simulink model "controller14"  (R2023a)
settings: Solver=FixedStepAuto  StartTime=0.0  StopTime=mdl.rt  RelTol=1e-3
values from neighbouring files (symbols this model uses):
  archived_Eul_XYZ = rst_Eul_XYZ.signals.values    [s4_run.m]    (also in step4_run_v1.m)
  archived_p_raw = rst_p_raw.signals.values    [s4_run.m]    (also in step4_run_v1.m)
  ctr = make_ext_tor_observer(rsim, mdl, ctr)    [s1_setup.m]    (also in setup_controller_with_functions.m = make_controller(); step1_setup.m; step1_setup_v1.m)
  ctr2 = ctr    [s1_setup.m]    (also in step1_setup.m; step1_setup_v1.m)
  lut = gen_lut    [s1_setup.m]    (also in thrust2voltage_lut_20230809.mat = ; thrust2voltage_lut_20230829.mat = )
  mdl = make_model(mdl,rsim)    [s1_setup.m]    (also in setup_controller_with_functions.m = make_model(flight_time); step1_setup.m; step1_setup_v1.m = make_model(flight_time,rsim))
  rbt = make_robot    [s1_setup.m]    (also in setup_controller_with_functions.m = make_robot(); step1_setup.m; step1_setup_v1.m)
  rbt2 = rbt    [s1_setup.m]    (also in step1_setup.m; step1_setup_v1.m)
  rsim = make_robot_simulation()    [setup_controller_with_functions.m]    (also in step1_setup_v1.m = make_simulation(rbt,mdl,rsim))
  som = make_somersault(mdl, rsim)    [s1_setup.m]    (also in step1_setup.m = make_somersault(mdl))
  traj = make_trajectory(ctr, mdl, rsim)    [s1_setup.m]    (also in step1_setup.m)
undefined symbols (not defined in the file or in its folder): DiscIntNeverNeededParam, Standard_Devices, UDP_Protocol
libraries: simulink x27, dspfdesign x7, robotcorelib x6, sldrtlib x4, slrealtimeloglib x1, shared6dof x1, dspsrcs4 x1, uavutilslib x1
(part 1 of 3)
settings Model: SimulationMode=external  ExtModeTrigDuration=5000000  Creator=SMRL  LastModifiedBy=SMRL
settings HardwareCC: ProdBitPerLong=64  ProdHWDeviceType=Intel->x86-64 (Linux 64)
settings RTWCC: Description=Simulink Desktop Real-Time  SystemTargetFile=sldrt.tlc  TemplateMakefile=sldrt.tmf  RTWCompilerOptimization=on
settings CodeAppCC: MaxIdLength=95
settings SimulinkDesktopRealTimeCC: TargetLibSuffix=_sldrt.a  TargetPreCompLibLocation=C:\Program Files\MATLAB\R2023a\toolbox\sldrt\lib\win64

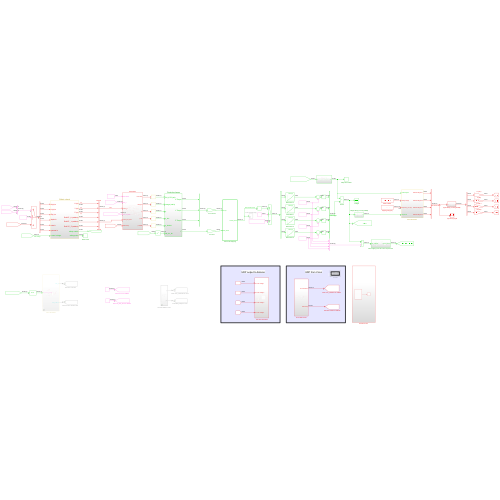
[thumbnail: Simulink's stored preview of the top-level diagram]
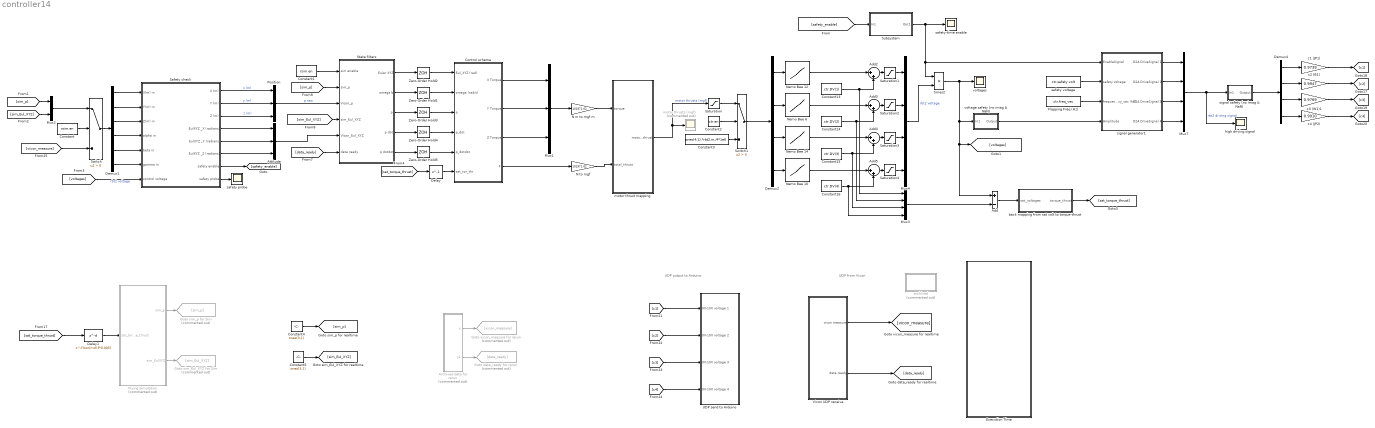
== system controller14 ==
  note: UDP output to Arduino
  note: UDP from Vicon
  Add : Sum  Inputs=+-
  Add{2..5} (4 alike) : Sum  Inputs=|++
  Archived data for rerun : Subsystem  Commented=on
  Attitude : Mux  Inputs=3
  Constant : Constant  Value=rsim.en
  Constant1 : Constant  Value=rsim.en
  Constant13 : Constant  Value=ctr.DV(1)
  Constant14 : Constant  Value=ctr.DV(2)
  Constant15 : Constant  Value=ctr.DV(3)
  Constant16 : Constant  Value=ctr.DV(4)
  Constant2 : Constant  Value=ctr.en
  Constant3 : Constant  Value=ones(4,1).*rbt2.m./4*1e6
  Constant4 : Constant  Value=ones(3,1)
  Constant5 : Constant  Value=ones(3,1)
  Control scheme : Subsystem
  Delay : Delay  DelayLength=1  InitialCondition=zeros(4,1)
  Delay1 : Delay  DelayLength=floor(mdl.f*0.005)  InitialCondition=zeros(4,floor(mdl.f*0.005))  SampleTime=mdl.T
  Demux1 : Demux  Outputs=6
  Demux2 : Demux
  Demux4 : Demux
  Execution Time : Subsystem
  Flapping Freq (Hz) : Constant  Value=ctr.freq_vec  VectorParams1D=off  SampleTime=mdl.T_high
  Flying Simulation : Subsystem  Commented=on
  Goto data_ready for rerun : Goto  Commented=on  GotoTag=data_ready
  Goto sim_Eul_XYZ for Sim : Goto  Commented=on  GotoTag=sim_Eul_XYZ
  Goto sim_p for Sim : Goto  Commented=on  GotoTag=sim_p
  Goto vicon_measure for rerun : Goto  Commented=on  GotoTag=vicon_measure
  Mux1 : Mux  Inputs=3
  Mux2 : Mux  Inputs=2
  Mux3 : Mux
  Mux4 : Mux
  Mux7 : Mux
  N m to mgf m : Gain  Gain=101971.62
  N to mgf : Gain  Gain=101971.62
  Nemo Bee 10 : Lookup_n-D  NumberOfTableDimensions=1  BreakpointsForDimension1=lut.T4  Table=lut.v4  InternalRulePriority=Speed  RndMeth=Simplest
  Nemo Bee 12 : Lookup_n-D  NumberOfTableDimensions=1  BreakpointsForDimension1=lut.T1  Table=lut.v1  InternalRulePriority=Speed  RndMeth=Simplest
  Nemo Bee 14 : Lookup_n-D  NumberOfTableDimensions=1  BreakpointsForDimension1=lut.T3  Table=lut.v3  InternalRulePriority=Speed  RndMeth=Simplest
  Nemo Bee 6 : Lookup_n-D  NumberOfTableDimensions=1  BreakpointsForDimension1=lut.T2  Table=lut.v2  InternalRulePriority=Speed  RndMeth=Simplest
  Position : Mux  Inputs=3
  Safety check : Subsystem  SystemSampleTime=mdl.T
  Saturation : Saturate  UpperLimit=1000  LowerLimit=0
  Saturation1 : Saturate  UpperLimit=ctr.safety.volt(1)  LowerLimit=0
  Saturation2 : Saturate  UpperLimit=ctr.safety.volt(2)  LowerLimit=0
  Saturation3 : Saturate  UpperLimit=ctr.safety.volt(3)  LowerLimit=0
  Saturation4 : Saturate  UpperLimit=ctr.safety.volt(4)  LowerLimit=0
  State filters : Subsystem
  Subsystem : Subsystem
  Switch : Switch  Criteria=u2 > Threshold  SaturateOnIntegerOverflow=off  InputSameDT=off
  Switch1 : Switch  Criteria=u2 > Threshold  SaturateOnIntegerOverflow=off  InputSameDT=off
  UDP send to Arduino : Subsystem
  Vicon UDP receive : Subsystem
  Zero-Order Hold{1..5} (5 alike) : ZeroOrderHold  SampleTime=mdl.T
  archived : Subsystem  Commented=on
  back mapping from sat volt to torque-thrust : Subsystem
  c1 (JP1) : Gain  Gain=0.9739
  c2 (B1) : Gain  Gain=0.9947
  c3 (W1)1 : Gain  Gain=0.9769
  c4 (JP2) : Gain  Gain=0.9910
  high driving signal : Scope
  motor thrust mapping : MATLAB Function  TreatAsAtomicUnit=on  SystemSampleTime=mdl.T
  motor thrusts (mgf) : Scope  Commented=on
  safety probe : Scope
  safety voltage : Constant  Value=ctr.safety.volt  SampleTime=mdl.T_high
  safety-time enable : Scope
  signal generator1 : Subsystem  SystemSampleTime=mdl.T_high
  signal safety (no imag & NaN) : Subsystem
  times2 : Product  RndMeth=Zero
  voltage safety (no imag & NaN) : Subsystem
  voltages : Scope
  wires:
  c3 (W1)1/1 -> [c3]
  c4 (JP2)/1 -> [c4]
  safety voltage/1 -> signal generator1/2(safety voltage)
  Demux4/4 -> c4 (JP2)/1
  signal safety (no imag & NaN)/1(Output) -> Demux4/1
  Safety check/3(Z (m)) -> Position/3  "z (m)"
  Demux4/3 -> c3 (W1)1/1
  Demux4/2 -> c2 (B1)/1
  voltage safety (no imag & NaN)/1(Output) -> signal generator1/4(Amplitude)
  Demux1/4 -> Safety check/4(alpha in)
  Safety check/2(Y (m)) -> Position/2  "y (m)"
  Saturation1/1 -> Mux4/1
  Saturation3/1 -> Mux4/3
  motor thrust mapping/1(motors_thrust) -> Saturation/1, motor thrusts (mgf)/1  "motor thrusts (mgf)"
  Demux4/1 -> c1 (JP1)/1
  Saturation2/1 -> Mux4/2
  Saturation4/1 -> Mux4/4
  Demux1/3 -> Safety check/3(Z(m) in)
  Demux1/2 -> Safety check/2(Y(m) in)
  signal generator1/1(D2A DriveSignal 1) -> Mux7/1
  Safety check/1(X (m)) -> Position/1  "x (m)"
  Mux7/1 -> signal safety (no imag & NaN)/1(In1), high driving signal/1  "rbt2 driving signal"
  c2 (B1)/1 -> [c2]
  Demux1/1 -> Safety check/1(X(m) in)
  c1 (JP1)/1 -> [c1]
  Demux1/6 -> Safety check/6(gamma in)
  signal generator1/2(D2A DriveSignal 2) -> Mux7/2
  signal generator1/3(D2A DriveSignal 3) -> Mux7/3
  Demux1/5 -> Safety check/5(beta in)
  Mux4/1 -> times2/2  "rbt2 voltage"
  Flapping Freq (Hz)/1 -> signal generator1/3(frequency_vec (hz))
  signal generator1/4(D2A DriveSignal 4) -> Mux7/4
  Safety check/6(EulXYZ _Z (radians)) -> Attitude/3
  Safety check/5(EulXYZ _Y (radians)) -> Attitude/2
  Safety check/4(EulXYZ _X (radians)) -> Attitude/1
  Vicon UDP receive/1(vicon measure) -> [vicon_measure]
  Vicon UDP receive/2(data ready) -> [data_ready]
  [c1] -> UDP send to Arduino/1(0V-10V voltage 1)
  [c2] -> UDP send to Arduino/2(0V-10V voltage 2)
  [c3] -> UDP send to Arduino/3(0V-10V voltage 3)
  [c4] -> UDP send to Arduino/4(0V-10V voltage 4)
  Safety check/7(safety enable) -> [safety_enable]
  Control scheme/1(X Torque) -> Mux1/1
  Control scheme/2(Y Torque) -> Mux1/2
  Control scheme/3(Z Torque) -> Mux1/3
  [sat_torque_thrust] -> Delay1/1
  Flying Simulation/2(sim_EulXYZ) -> Goto sim_Eul_XYZ for Sim/1
  Flying Simulation/1(sim_p) -> Goto sim_p for Sim/1
  [sim_p] -> Mux2/1
  [sim_Eul_XYZ] -> Mux2/2
  Constant/1 -> Switch/2
  Mux2/1 -> Switch/1
  [vicon_measure] -> Switch/3
  Switch/1 -> Demux1/1
  State filters/1(Euler XYZ) -> Zero-Order Hold2/1
  State filters/2(omega b) -> Zero-Order Hold1/1
  [sim_p] -> State filters/2(sim_p)
  [data_ready] -> State filters/6(data ready)
  State filters/3("p ") -> Zero-Order Hold3/1
  State filters/4(p dot) -> Zero-Order Hold4/1
  Position/1 -> State filters/3(Vicon_p)  "p raw"
  Constant1/1 -> State filters/1(sim enable)
  Attitude/1 -> State filters/5(Vicon_Eul_XYZ)
  [sim_Eul_XYZ] -> State filters/4(sim_Eul_XYZ)
  Zero-Order Hold2/1 -> Control scheme/1(Eul_XYZ (rad))
  Zero-Order Hold1/1 -> Control scheme/2(omega (rad/s))
  Zero-Order Hold3/1 -> Control scheme/3(p)
  Zero-Order Hold4/1 -> Control scheme/4(p_dot)
  Zero-Order Hold5/1 -> Control scheme/5(p_dotdot)
  State filters/5(p dotdot) -> Zero-Order Hold5/1
  N m to mgf m/1 -> motor thrust mapping/1(torque)
  N to mgf/1 -> motor thrust mapping/2(total_thrust)
  Constant14/1 -> Mux3/2, Add3/2
  Constant15/1 -> Mux3/3, Add4/2
  Constant16/1 -> Mux3/4, Add5/2
  Nemo Bee 6/1 -> Add3/1
  Nemo Bee 14/1 -> Add4/1
  Nemo Bee 12/1 -> Add2/1
  Nemo Bee 10/1 -> Add5/1
  Constant13/1 -> Mux3/1, Add2/2
  Add3/1 -> Saturation2/1
  Add2/1 -> Saturation1/1
  Add4/1 -> Saturation3/1
  Add5/1 -> Saturation4/1
  Demux2/1 -> Nemo Bee 12/1
  Demux2/2 -> Nemo Bee 6/1
  Demux2/3 -> Nemo Bee 14/1
  Demux2/4 -> Nemo Bee 10/1
  Constant2/1 -> Switch1/2
  Saturation/1 -> Switch1/1
  Switch1/1 -> Demux2/1
  Constant3/1 -> Switch1/3
  times2/1 -> voltage safety (no imag & NaN)/1(In1), [voltages], Add/1, voltages/1
  Constant4/1 -> [sim_p]
  Constant5/1 -> [sim_Eul_XYZ]
  [voltages] -> Safety check/7(control voltage)  "rbt2 voltage"
  Archived data for rerun/1(y) -> Goto vicon_measure for rerun/1
  Archived data for rerun/2(y1) -> Goto data_ready for rerun/1
  Mux3/1 -> Add/2
  Add/1 -> back mapping from sat volt to torque-thrust/1(sat_voltages)
  back mapping from sat volt to torque-thrust/1(torque_thrust) -> [sat_torque_thrust]
  Control scheme/4(" F") -> N to mgf/1
  Mux1/1 -> N m to mgf m/1
  Subsystem/1(Out1) -> signal generator1/1(EnableSignal), times2/1, safety-time enable/1
  [safety_enable] -> Subsystem/1(In1)
  Safety check/8(safety probe) -> safety probe/1
  [sat_torque_thrust] -> Delay/1
  Delay/1 -> Control scheme/6(sat_tor_thr)
  Delay1/1 -> Flying Simulation/1(sat_torque_thrust)

== system controller14/Archived data for rerun ==
  MATLAB Function1 : MATLAB Function  TreatAsAtomicUnit=on
  MATLAB Function2 : MATLAB Function  TreatAsAtomicUnit=on
  Scope1 : Scope
  Scope2 : Scope
  Scope3 : Scope
  time1 : Subsystem
  y : Outport
  y1 : Outport  Port=2
  wires:
  MATLAB Function2/1(y) -> y/1, Scope1/1
  time1/1(index) -> Scope2/1, MATLAB Function2/1(t), MATLAB Function1/1(t)
  MATLAB Function1/1(y) -> y1/1, Scope3/1

== system controller14/Control scheme ==
  Eul_XYZ (rad) : Inport
  omega (rad/s) : Inport  Port=2
  p : Inport  Port=3
  p_dot : Inport  Port=4
  p_dotdot : Inport  Port=5
  sat_tor_thr : Inport  Port=6
  Coordinate Transformation Conversion : robotcorelib/Coordinate Transformation Conversion  InputRepresentation=Euler Angles  InputEulerSequence=XYZ  ShowTrVecInputPort=on  OutputRepresentation=Rotation Matrix  OutputEulerSequence=ZYX  ShowTrVecOutputPort=on  SimulateUsing=Interpreted execution
  Delay : Delay  DelayLength=1  InitialCondition=1
  Delay1 : Delay  DelayLength=1  InitialCondition=zeros(3,1)
  adaptive setpoint rd : MATLAB Function  TreatAsAtomicUnit=on  SystemSampleTime=mdl.T
  all states : Scope  NumInputPorts=4
  attitude and thrust controller : Subsystem
  observer : Subsystem  Commented=on
  p vs p_des : Scope  NumInputPorts=2
  saturation : MATLAB Function  TreatAsAtomicUnit=on
  time : Subsystem
  unsat thrust : Scope
  unsat torque : Scope  NumInputPorts=3
  X Torque : Outport
  Y Torque : Outport  Port=2
  Z Torque : Outport  Port=3
  " F" : Outport  Port=4
  wires:
  Eul_XYZ (rad)/1 -> Coordinate Transformation Conversion/1
  omega (rad/s)/1 -> all states/4, attitude and thrust controller/5(Omega)
  saturation/1(X_roll) -> X Torque/1
  saturation/2(Y_pitch) -> Y Torque/1
  saturation/3(Z_yaw) -> Z Torque/1
  saturation/4(Force) -> " F"/1
  attitude and thrust controller/4(F) -> saturation/4(F), unsat thrust/1
  adaptive setpoint rd/1(rd) -> p vs p_des/2, attitude and thrust controller/6(rd)  "rd"
  adaptive setpoint rd/2(rd_d) -> attitude and thrust controller/7(rd_d)
  adaptive setpoint rd/3(rd_dd) -> attitude and thrust controller/8(rd_dd)
  adaptive setpoint rd/4(rd_ddd) -> attitude and thrust controller/9(rd_ddd)
  adaptive setpoint rd/5(rd_dddd) -> attitude and thrust controller/10(rd_dddd)
  time/1(real times) -> adaptive setpoint rd/2(time)
  attitude and thrust controller/3(torque_z) -> saturation/3(z_yaw), unsat torque/3
  attitude and thrust controller/2(torque_y) -> saturation/2(y_pitch), unsat torque/2
  attitude and thrust controller/1(torque_x) -> unsat torque/1, saturation/1(x_roll)
  adaptive setpoint rd/7(id_out) -> Delay/1
  Delay/1 -> adaptive setpoint rd/4(id_in)
  Coordinate Transformation Conversion/1 -> all states/3, attitude and thrust controller/4(R)  "rotm"
  p_dot/1 -> all states/2, attitude and thrust controller/2(r_dot)
  p_dotdot/1 -> attitude and thrust controller/3(r_dotdot)
  p/1 -> adaptive setpoint rd/1(r), p vs p_des/1, attitude and thrust controller/1(r), all states/1
  adaptive setpoint rd/6(init_r_out) -> Delay1/1
  Delay1/1 -> adaptive setpoint rd/3(init_r_in)
  sat_tor_thr/1 -> attitude and thrust controller/11(sat_tor_thr)

== system controller14/Execution Time ==
  Execution Time : sldrtlib/Target Profiling/Execution Time  ShowTaskTimes=off
  high execution time : Scope
  wires:
  Execution Time/1 -> high execution time/1

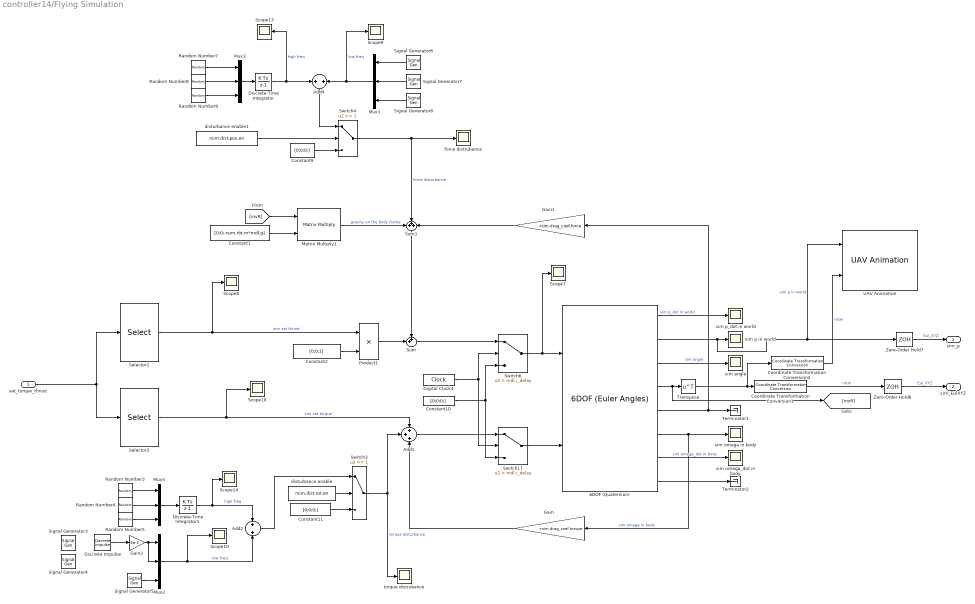
== system controller14/Flying Simulation ==
  sat_torque_thrust : Inport
  6DOF (Quaternion) : shared6dof/6DOF (Euler Angles)  units=Metric (MKS)  mtype=Fixed  rep=Quaternion  xme_0=rsim.p0  Vm_0=rsim.v0_b  eul_0=[rsim.Eul_XYZ.x rsim.Eul_XYZ.y rsim.Eul_XYZ.z]  pm_0=rsim.w0  mass_0=rsim.rbt.m  mass_e=0.5  mass_f=2.0  inertia=diag([rsim.rbt.ixx, rsim.rbt.iyy, rsim.rbt.izz])  inertia_e=eye(3)  inertia_f=2*eye(3)  k_quat=1.0  vre_flag=on  abi_flag=off  aMode=0  xme_statename=''  Vm_statename=''  eul_statename=''  quat_statename=''  pm_statename=''  mass_statename=''
      settings: LibrarySourceBlock=aerolib6dof2/6DOF (Quaternion)
  Add1 : Sum  Inputs=+++
  Add2 : Sum
  Add4 : Sum
  Constant1 : Constant  Value=[0;0;-rsim.rbt.m*mdl.g]
  Constant10 : Constant  Value=[0;0;0;]
  Constant11 : Constant  Value=[0;0;0;]
  Constant2 : Constant  Value=[0;0;1]
  Constant9 : Constant  Value=[0;0;0;]
  Coordinate Transformation Conversion1 : robotcorelib/Coordinate Transformation Conversion  InputRepresentation=Rotation Matrix  InputEulerSequence=XYZ  ShowTrVecInputPort=on  OutputRepresentation=Euler Angles  OutputEulerSequence=XYZ  ShowTrVecOutputPort=on  SimulateUsing=Interpreted execution
  Coordinate Transformation Conversion2 : robotcorelib/Coordinate Transformation Conversion  InputRepresentation=Rotation Matrix  InputEulerSequence=XYZ  ShowTrVecInputPort=on  OutputRepresentation=Quaternion  OutputEulerSequence=XYZ  ShowTrVecOutputPort=on  SimulateUsing=Interpreted execution
  Digital Clock4 : DigitalClock  SampleTime=1/2000
  Discrete Impulse : dspsrcs4/Discrete  Impulse  Delay=mdl.f*3.1  SampleTime=mdl.T  FrameSample=1  OutputFrames=off  dataType=double  isSigned=on  wordLen=16  udDataType=sfix(16)  fracBitsMode=Best precision  numFracBits=15  OutDataTypeStr=double  LastOutDataTypeStr=double
  Discrete-Time Integrator : DiscreteIntegrator  InitialCondition=[rsim.dist.x.mean; rsim.dist.y.mean; rsim.dist.z.mean]  SampleTime=mdl.T  ICPrevOutput=DiscIntNeverNeededParam  ICPrevScaledInput=DiscIntNeverNeededParam
  Discrete-Time Integrator1 : DiscreteIntegrator  InitialCondition=[rsim.dist.wx.mean; rsim.dist.wy.mean; rsim.dist.wz.mean]  SampleTime=mdl.T  ICPrevOutput=DiscIntNeverNeededParam  ICPrevScaledInput=DiscIntNeverNeededParam
  Gain : Gain  Gain=-rsim.drag_coef.torque
  Gain1 : Gain  Gain=-rsim.drag_coef.force
  Gain2 : Gain  Gain=5e-3
  Matrix Multiply1 : Product  Multiplication=Matrix(*)
  Mux{1..3,5} (4 alike) : Mux  Inputs=3
  Product1 : Product
  Random Number3 : RandomNumber  Variance=rsim.dist.wx.var  Seed=rsim.dist.wx.seed  SampleTime=1/2000
  Random Number4 : RandomNumber  Variance=rsim.dist.wy.var  Seed=rsim.dist.wy.seed  SampleTime=1/2000
  Random Number5 : RandomNumber  Variance=rsim.dist.wz.var  Seed=rsim.dist.wz.seed  SampleTime=1/2000
  Random Number7 : RandomNumber  Variance=rsim.dist.x.var  Seed=rsim.dist.x.seed  SampleTime=mdl.T
  Random Number8 : RandomNumber  Variance=rsim.dist.y.var  Seed=rsim.dist.y.seed  SampleTime=mdl.T
  Random Number9 : RandomNumber  Variance=rsim.dist.z.var  Seed=rsim.dist.z.seed  SampleTime=mdl.T
  Scope{7..10,13..14,19} (7 alike) : Scope
  Selector1 : Selector  InputPortWidth=4  IndexOptions=Index vector (dialog)  Indices=[4]  OutputSizes=1
  Selector2 : Selector  InputPortWidth=4  IndexOptions=Index vector (dialog)  Indices=[1:3]  OutputSizes=1
  Signal Generator3 : SignalGenerator  WaveForm=square  Amplitude=2e-5  Frequency=0.1618
  Signal Generator4 : SignalGenerator  WaveForm=square  Amplitude=0e-5  Frequency=0.162
  Signal Generator5 : SignalGenerator  Amplitude=-30e-8  Frequency=0.4
  Signal Generator6 : SignalGenerator  WaveForm=square  Amplitude=0  Frequency=0.1
  Signal Generator7 : SignalGenerator  WaveForm=square  Amplitude=0  Frequency=0.5
  Signal Generator8 : SignalGenerator  WaveForm=square  Amplitude=0  Frequency=0.5
  Sum : Sum  Inputs=++|
  Sum1 : Sum  Inputs=+++
  Switch17 : Switch  Criteria=u2 > Threshold  Threshold=mdl.i_delay  SaturateOnIntegerOverflow=off  InputSameDT=off
  Switch3 : Switch  Threshold=1  SaturateOnIntegerOverflow=off  InputSameDT=off
  Switch4 : Switch  Threshold=1  SaturateOnIntegerOverflow=off  InputSameDT=off
  Switch6 : Switch  Criteria=u2 > Threshold  Threshold=mdl.i_delay  SaturateOnIntegerOverflow=off  InputSameDT=off
  Terminator1 : Terminator
  Terminator2 : Terminator
  Transpose : Math  Operator=transpose  SignedPower=on
  UAV Animation : uavutilslib/UAV Animation  UAVType=Multirotor  UAVSize=0.1  InertialZDirection=Up  SampleTime=1/100
  Zero-Order Hold6 : ZeroOrderHold  SampleTime=1/400
  Zero-Order Hold7 : ZeroOrderHold  SampleTime=1/400
  disturbance enable : Constant  Value=rsim.dist.rot.en
  disturbance enable1 : Constant  Value=rsim.dist.pos.en
  force distrubance : Scope
  sim angle : Scope
  sim omega in body : Scope
  sim omega_dot in body : Scope
  sim p in world : Scope
  sim p_dot in world : Scope
  torque distrubance : Scope
  sim_p : Outport
  sim_EulXYZ : Outport  Port=2
  wires:
  Random Number5/1 -> Mux5/3
  disturbance enable/1 -> Switch3/2
  Mux5/1 -> Discrete-Time Integrator1/1
  Digital Clock4/1 -> Switch6/2, Switch17/2
  Constant11/1 -> Switch3/3
  Constant2/1 -> Product1/2
  Constant1/1 -> Matrix Multiply1/2
  Random Number3/1 -> Mux5/1
  Matrix Multiply1/1 -> Sum1/1  "gravity on the body frame"
  disturbance enable1/1 -> Switch4/2
  Random Number4/1 -> Mux5/2
  Switch3/1 -> Add1/2, torque distrubance/1  "torque disturbance"
  Constant9/1 -> Switch4/3
  [invR] -> Matrix Multiply1/1
  Constant10/1 -> Switch6/3, Switch17/3
  Sum1/1 -> Sum/1
  Sum/1 -> Switch6/1
  Switch4/1 -> Sum1/2, force distrubance/1  "force disturbance"
  Product1/1 -> Sum/2
  Add1/1 -> Switch17/1
  Switch6/1 -> Scope7/1, 6DOF (Quaternion)/1
  Switch17/1 -> 6DOF (Quaternion)/2
  6DOF (Quaternion)/1 -> sim p_dot in world/1  "sim p_dot in world"
  6DOF (Quaternion)/2 -> UAV Animation/1, Zero-Order Hold7/1, sim p in world/1  "sim p in world"
  6DOF (Quaternion)/3 -> sim angle/1  "sim angle"
  6DOF (Quaternion)/4 -> [invR], Transpose/1
  6DOF (Quaternion)/5 -> Gain1/1, Terminator1/1
  6DOF (Quaternion)/6 -> Gain/1, sim omega in body/1  "sim omega in body"
  6DOF (Quaternion)/7 -> sim omega_dot in body/1  "sim omega_dot in body"
  6DOF (Quaternion)/8 -> Terminator2/1
  Transpose/1 -> Coordinate Transformation Conversion2/1, Coordinate Transformation Conversion1/1
  Zero-Order Hold6/1 -> sim_EulXYZ/1  "Eul_XYZ"
  Coordinate Transformation Conversion1/1 -> Zero-Order Hold6/1  "rotm"
  Zero-Order Hold7/1 -> sim_p/1  "Eul_XYZ"
  Mux2/1 -> Scope10/1, Add2/2  "low freq"
  Signal Generator5/1 -> Mux2/3
  sat_torque_thrust/1 -> Selector1/1, Selector2/1
  Selector1/1 -> Scope8/1, Product1/1  "sim sat thrust"
  Selector2/1 -> Scope19/1, Add1/1  "sim sat torque"
  Random Number7/1 -> Mux3/1
  Mux3/1 -> Discrete-Time Integrator/1
  Random Number8/1 -> Mux3/2
  Random Number9/1 -> Mux3/3
  Discrete-Time Integrator/1 -> Add4/1, Scope13/1  "high freq"
  Mux1/1 -> Scope9/1, Add4/2  "low freq"
  Signal Generator8/1 -> Mux1/3
  Signal Generator7/1 -> Mux1/2
  Signal Generator6/1 -> Mux1/1
  Add4/1 -> Switch4/1
  Discrete-Time Integrator1/1 -> Add2/1, Scope14/1  "high freq"
  Add2/1 -> Switch3/1
  Coordinate Transformation Conversion2/1 -> UAV Animation/2  "rotm"
  Gain/1 -> Add1/3
  Gain1/1 -> Sum1/3
  Discrete Impulse/1 -> Gain2/1
  Gain2/1 -> Mux2/2, Mux2/1

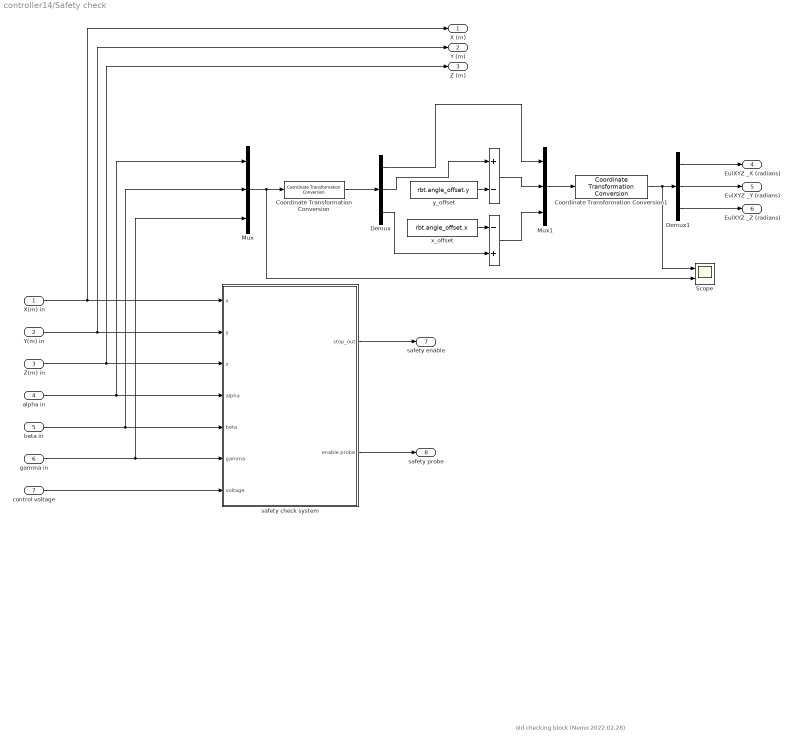
== system controller14/Safety check ==
  note: old checking block (Nemo 2022.02.28)
  X(m) in : Inport
  Y(m) in : Inport  Port=2
  Z(m) in : Inport  Port=3
  alpha in : Inport  Port=4
  beta in : Inport  Port=5
  gamma in : Inport  Port=6
  control voltage : Inport  Port=7
  " " : Sum  Inputs=-+
  "  " : Sum  Inputs=+-
  Coordinate Transformation Conversion : robotcorelib/Coordinate Transformation Conversion  InputRepresentation=Euler Angles  InputEulerSequence=XYZ  ShowTrVecInputPort=on  OutputRepresentation=Euler Angles  OutputEulerSequence=ZYX  ShowTrVecOutputPort=on  SimulateUsing=Interpreted execution
  Coordinate Transformation Conversion1 : robotcorelib/Coordinate Transformation Conversion  InputRepresentation=Euler Angles  InputEulerSequence=ZYX  ShowTrVecInputPort=on  OutputRepresentation=Euler Angles  OutputEulerSequence=XYZ  ShowTrVecOutputPort=on  SimulateUsing=Interpreted execution
  Demux : Demux  Outputs=3
  Demux1 : Demux  Outputs=3
  Mux : Mux  Inputs=3
  Mux1 : Mux  Inputs=3
  Scope : Scope  NumInputPorts=2
  safety check system : Subsystem
  x_offset : Constant  Value=rbt.angle_offset.x
  y_offset : Constant  Value=rbt.angle_offset.y
  X (m) : Outport
  Y (m) : Outport  Port=2
  Z (m) : Outport  Port=3
  EulXYZ _X (radians) : Outport  Port=4
  EulXYZ _Y (radians) : Outport  Port=5
  EulXYZ _Z (radians) : Outport  Port=6
  safety enable : Outport  Port=7
  safety probe : Outport  Port=8
  wires:
  X(m) in/1 -> X (m)/1, safety check system/1(x)
  Y(m) in/1 -> Y (m)/1, safety check system/2(y)
  Z(m) in/1 -> Z (m)/1, safety check system/3(z)
  alpha in/1 -> Mux/1, safety check system/4(alpha)
  beta in/1 -> Mux/2, safety check system/5(beta)
  y_offset/1 -> "  "/2
  control voltage/1 -> safety check system/7(voltage)
  safety check system/1(stop_out) -> safety enable/1
  gamma in/1 -> Mux/3, safety check system/6(gamma)
  Mux/1 -> Scope/2, Coordinate Transformation Conversion/1
  Coordinate Transformation Conversion/1 -> Demux/1
  Demux/2 -> "  "/1
  "  "/1 -> Mux1/2
  Mux1/1 -> Coordinate Transformation Conversion1/1
  Coordinate Transformation Conversion1/1 -> Scope/1, Demux1/1
  Demux1/1 -> EulXYZ _X (radians)/1
  Demux1/2 -> EulXYZ _Y (radians)/1
  Demux1/3 -> EulXYZ _Z (radians)/1
  safety check system/2(enable probe) -> safety probe/1
  Demux/1 -> Mux1/1
  x_offset/1 -> " "/1
  " "/1 -> Mux1/3
  Demux/3 -> " "/2

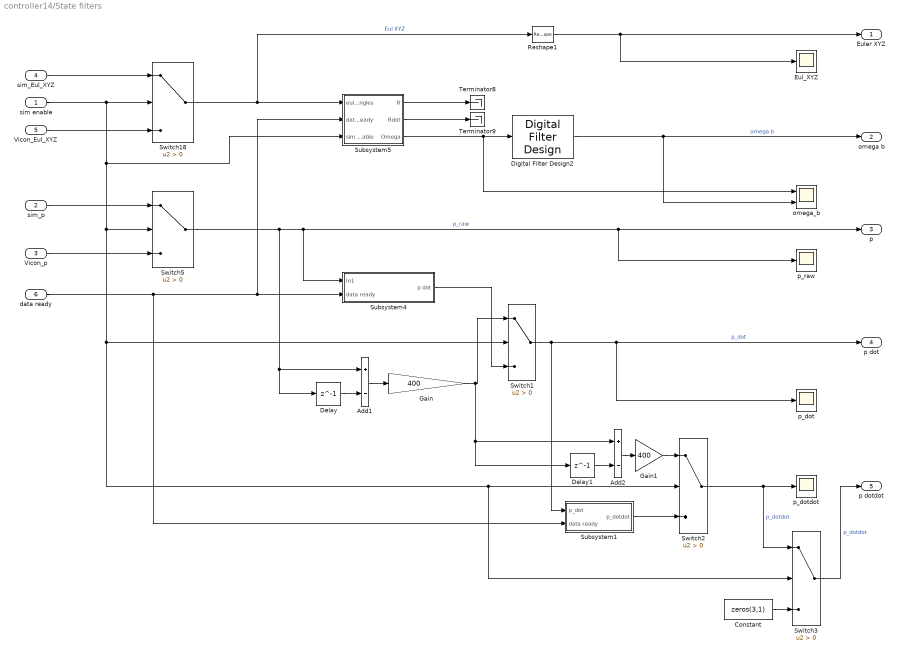
== system controller14/State filters ==
  sim enable : Inport
  sim_p : Inport  Port=2
  Vicon_p : Inport  Port=3
  sim_Eul_XYZ : Inport  Port=4
  Vicon_Eul_XYZ : Inport  Port=5
  data ready : Inport  Port=6
  Add1 : Sum  Inputs=+-
  Add2 : Sum  Inputs=+-
  Constant : Constant  Value=zeros(3,1)
  Delay : Delay  DelayLength=1  InitialCondition=zeros(3,1)
  Delay1 : Delay  DelayLength=1  InitialCondition=zeros(3,1)
  Digital Filter Design2 : dspfdesign/Digital Filter Design  mwdsp_browser_bugfix_var=off
  Eul_XYZ : Scope
  Gain : Gain  Gain=400
  Gain1 : Gain  Gain=400
  Reshape1 : Reshape
  Subsystem1 : Subsystem
  Subsystem4 : Subsystem
  Subsystem5 : Subsystem
  Switch{1..3,5,18} (5 alike) : Switch  Criteria=u2 > Threshold  SaturateOnIntegerOverflow=off  InputSameDT=off
  Terminator8 : Terminator
  Terminator9 : Terminator
  omega_b : Scope  NumInputPorts=2
  p_dot : Scope
  p_dotdot : Scope
  p_raw : Scope
  Euler XYZ : Outport
  omega b : Outport  Port=2
  "p " : Outport  Port=3
  p dot : Outport  Port=4
  p dotdot : Outport  Port=5
  wires:
  Digital Filter Design2/1 -> omega b/1, omega_b/2  "omega b"
  Switch5/1 -> Delay/1, Add1/1, Subsystem4/1(In1), "p "/1, p_raw/1  "p_raw"
  Switch18/1 -> Reshape1/1, Subsystem5/1(euler_angles)  "Eul XYZ"
  Subsystem5/1(R) -> Terminator8/1
  sim enable/1 -> Subsystem5/3(sim enable), Switch3/2, Switch2/2, Switch1/2, Switch5/2, Switch18/2
  Subsystem5/3(Omega) -> omega_b/1, Digital Filter Design2/1
  Vicon_p/1 -> Switch5/3
  Subsystem5/2(Rdot) -> Terminator9/1
  Vicon_Eul_XYZ/1 -> Switch18/3
  data ready/1 -> Subsystem1/2(data ready), Subsystem4/2(data ready), Subsystem5/2(data ready)
  sim_p/1 -> Switch5/1
  sim_Eul_XYZ/1 -> Switch18/1
  Delay/1 -> Add1/2
  Add1/1 -> Gain/1
  Gain/1 -> Delay1/1, Add2/1, Switch1/1
  Subsystem4/1(p dot) -> Switch1/3
  Switch1/1 -> p_dot/1, p dot/1, Subsystem1/1(p_dot)  "p_dot"
  Add2/1 -> Gain1/1
  Delay1/1 -> Add2/2
  Subsystem1/1(p_dotdot) -> Switch2/3
  Gain1/1 -> Switch2/1
  Switch2/1 -> Switch3/1, p_dotdot/1  "p_dotdot"
  Reshape1/1 -> Eul_XYZ/1, Euler XYZ/1
  Constant/1 -> Switch3/3
  Switch3/1 -> p dotdot/1  "p_dotdot"

== system controller14/Subsystem ==
  In1 : Inport
  Constant8 : Constant
  Constant9 : Constant  Value=rsim.en
  Data Type Conversion1 : DataTypeConversion  SaturateOnIntegerOverflow=off  RndMeth=Floor
  MATLAB Function : MATLAB Function  TreatAsAtomicUnit=on
  Switch2 : Switch  Criteria=u2 > Threshold  SaturateOnIntegerOverflow=off  InputSameDT=off
  Zero-Order Hold6 : ZeroOrderHold  SampleTime=mdl.T
  time : Subsystem
  times1 : Product  RndMeth=Zero
  Out1 : Outport
  wires:
  Constant9/1 -> Switch2/2
  Switch2/1 -> times1/1
  Constant8/1 -> Data Type Conversion1/1
  time/1(real times) -> MATLAB Function/1(t)
  times1/1 -> Zero-Order Hold6/1
  MATLAB Function/1(enable) -> times1/2
  In1/1 -> Switch2/3
  Data Type Conversion1/1 -> Switch2/1
  Zero-Order Hold6/1 -> Out1/1

== system controller14/UDP send to Arduino ==
  0V-10V voltage 1 : Inport
  0V-10V voltage 2 : Inport  Port=2
  0V-10V voltage 3 : Inport  Port=3
  0V-10V voltage 4 : Inport  Port=4
  Digital Clock : DigitalClock  SampleTime=1/10000
  Packet Output : sldrtlib/Packet Output  SampleTime=1/10000  MaxMissedTicks=100  ShowMissedTicks=off  YieldWhenWaiting=off  DrvName=Standard_Devices/UDP_Protocol  DrvAddress=22099  DrvOptions=[0 25000 49 54 57 46 50 53 52 46 49 48 51 46 52 50 0 0 0 0 0 0 0 0 0 0 0 0 0 0 0 0 0 0 0 0 0 0 0 0 0 0 0 0 0 0 0 0 0 0 0 0 0 0 0 0 0 0 0 0 0 0 0 0 0 0 0 0 0 0 0 0 0 0 0 0 0 0 0 0 0 0 0 0 0 0 0 0 0 0 0 0 0 0 0 0 0 0 0 0 0 0 0 0 0 0 0 0 0 0 0 0 0 0 0 0 0 0 0 0 0 0 0 0 0 0 0 0 0 0 0 0 0 0 0 0 0 0 0 0 0 0 0 0 0 0 0 0 0 0 0 0 0 0 0 0 0 0 0 0 0 0 0 0 0 0 0 0 0 0 0 0 0 0 0 0 0 0 0 0 0 0 0 0 0 0 0 0 0 0 0 0 0 0 0 0 0 0 0 0 0 0 0 0 0 0 0 0 0 0 0 0 0 0 0 0 0 0 0 0 0 0 0 0 0 0 0 0 0 0 0 0 0 0 0 0 0 0 0 0 0 0 0 0 0 0 0 0 0 0 0 0 0 0 0 0]  PacketSize=8  DataTypes='4*uint16'  ShowReady=off  ShowError=off  PacketID=1  ByteOrder=1  InitialValue=[]  FinalValue=[]
      settings: AttributesFormatString=UDP Protocol [22099]
  Switch : Switch  Criteria=u2 > Threshold  Threshold=2  SaturateOnIntegerOverflow=off  InputSameDT=off
  UDP send to Arduino DAC : Subsystem
  constant1 : Constant  Value=0  OutDataTypeStr=boolean
  constant2 : Constant  OutDataTypeStr=boolean
  wires:
  UDP send to Arduino DAC/1(Output) -> Packet Output/1
  0V-10V voltage 2/1 -> UDP send to Arduino DAC/2(DAC2)
  0V-10V voltage 4/1 -> UDP send to Arduino DAC/4(DAC4)
  0V-10V voltage 1/1 -> UDP send to Arduino DAC/1(DAC1)
  Switch/1 -> UDP send to Arduino DAC/5(DO2)
  0V-10V voltage 3/1 -> UDP send to Arduino DAC/3(DAC3)
  constant1/1 -> Switch/1
  constant2/1 -> Switch/3
  Digital Clock/1 -> Switch/2

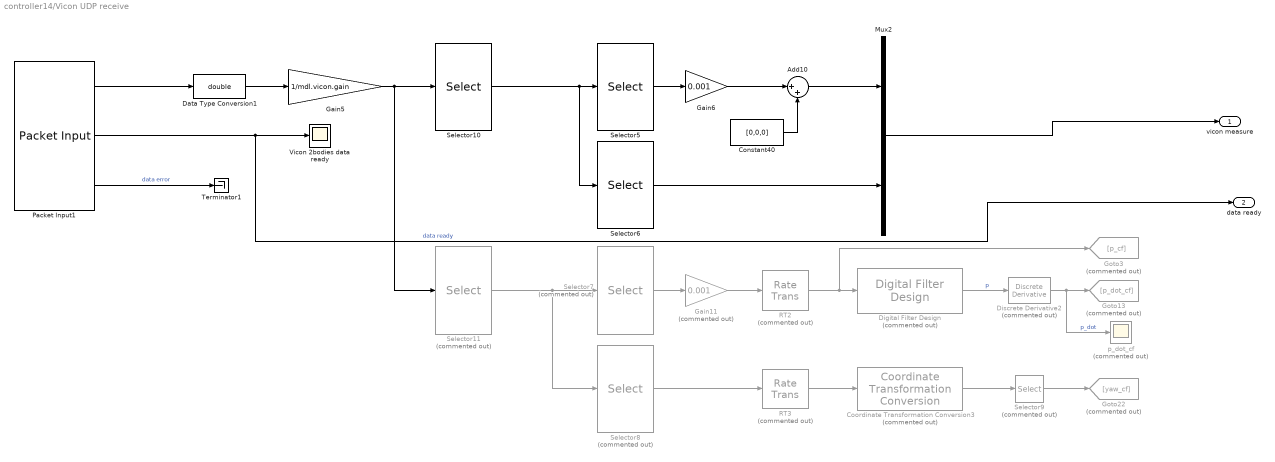
== system controller14/Vicon UDP receive ==
  Add10 : Sum  Inputs=|++
  Constant40 : Constant  Value=[0,0,0]
  Coordinate Transformation Conversion3 : robotcorelib/Coordinate Transformation Conversion  Commented=on  InputRepresentation=Euler Angles  InputEulerSequence=XYZ  ShowTrVecInputPort=on  OutputRepresentation=Euler Angles  OutputEulerSequence=ZYX  ShowTrVecOutputPort=on  SimulateUsing=Interpreted execution
  Data Type Conversion1 : DataTypeConversion  OutDataTypeStr=double  SaturateOnIntegerOverflow=off  RndMeth=Floor
  Digital Filter Design : dspfdesign/Digital Filter Design  Commented=on  mwdsp_browser_bugfix_var=off
  Discrete Derivative2 : simulink/Discrete/Discrete Derivative  Commented=on  gainval=1.0  ICPrevScaledInput=0.0  OutMin=[]  OutMax=[]  OutDataType=fixdt(1, 16)  OutScaling=2^-10  DoSatur=off
  Gain11 : Gain  Commented=on  Gain=0.001
  Gain5 : Gain  Gain=1/mdl.vicon.gain
  Gain6 : Gain  Gain=0.001
  Goto13 : Goto  Commented=on  GotoTag=p_dot_cf
  Goto22 : Goto  Commented=on  GotoTag=yaw_cf
  Goto3 : Goto  Commented=on  GotoTag=p_cf
  Mux2 : Mux  Inputs=2
  Packet Input1 : sldrtlib/Packet Input  SampleTime=1/10000  MaxMissedTicks=100  ShowMissedTicks=off  YieldWhenWaiting=off  DrvName=Standard_Devices/UDP_Protocol  DrvAddress=18000  DrvOptions=[0 18885 49 54 57 46 50 53 52 46 49 54 56 46 49 52 54 0 0 0 0 0 0 0 0 0 0 0 0 0 0 0 0 0 0 0 0 0 0 0 0 0 0 0 0 0 0 0 0 0 0 0 0 0 0 0 0 0 0 0 0 0 0 0 0 0 0 0 0 0 0 0 0 0 0 0 0 0 0 0 0 0 0 0 0 0 0 0 0 0 0 0 0 0 0 0 0 0 0 0 0 0 0 0 0 0 0 0 0 0 0 0 0 0 0 0 0 0 0 0 0 0 0 0 0 0 0 0 0 0 0 0 0 0 0 0 0 0 0 0 0 0 0 0 0 0 0 0 0 0 0 0 0 0 0 0 0 0 0 0 0 0 0 0 0 0 0 0 0 0 0 0 0 0 0 0 0 0 0 0 0 0 0 0 0 0 0 0 0 0 0 0 0 0 0 0 0 0 0 0 0 0 0 0 0 0 0 0 0 0 0 0 0 0 0 0 0 0 0 0 0 0 0 0 0 0 0 0 0 0 0 0 0 0 0 0 0 0 0 0 0 0 0 0 0 0 0 0 0 0 0 0 0 0 0 0]  PacketSize=48  DataTypes='12*int32'  ShowReady=on  ShowError=on  PacketID=1  ByteOrder=2  ShowTimestamp=off
      settings: AttributesFormatString=UDP Protocol [18000]
  RT2 : RateTransition  Commented=on  Integrity=off  OutPortSampleTime=1/100
  RT3 : RateTransition  Commented=on  Integrity=off  OutPortSampleTime=1/100
  Selector10 : Selector  InputPortWidth=12  IndexOptions=Index vector (dialog)  Indices=[1:6]  OutputSizes=1
  Selector11 : Selector  Commented=on  InputPortWidth=12  IndexOptions=Index vector (dialog)  Indices=[7:12]  OutputSizes=1
  Selector5 : Selector  InputPortWidth=6  IndexOptions=Index vector (dialog)  Indices=[1:3]  OutputSizes=1
  Selector6 : Selector  InputPortWidth=6  IndexOptions=Index vector (dialog)  Indices=[4:6]  OutputSizes=1
  Selector7 : Selector  Commented=on  InputPortWidth=6  IndexOptions=Index vector (dialog)  Indices=[1:3]  OutputSizes=1
  Selector8 : Selector  Commented=on  InputPortWidth=6  IndexOptions=Index vector (dialog)  Indices=[4:6]  OutputSizes=1
  Selector9 : Selector  Commented=on  InputPortWidth=3  IndexOptions=Index vector (dialog)  Indices=[1]  OutputSizes=1
  Terminator1 : Terminator
  Vicon 2bodies data ready : Scope
  p_dot_cf : Scope  Commented=on
  vicon measure : Outport
  data ready : Outport  Port=2
  wires:
  Gain5/1 -> Selector11/1, Selector10/1
  Selector9/1 -> Goto22/1
  Discrete Derivative2/1 -> Goto13/1, p_dot_cf/1  "p_dot"
  Selector11/1 -> Selector8/1, Selector7/1
  RT3/1 -> Coordinate Transformation Conversion3/1
  Gain11/1 -> RT2/1
  Packet Input1/2 -> data ready/1, Vicon 2bodies data ready/1  "data ready"
  Digital Filter Design/1 -> Discrete Derivative2/1  "p"
  Selector6/1 -> Mux2/2
  Coordinate Transformation Conversion3/1 -> Selector9/1
  Selector5/1 -> Gain6/1
  Selector10/1 -> Selector6/1, Selector5/1
  Data Type Conversion1/1 -> Gain5/1
  Selector7/1 -> Gain11/1
  RT2/1 -> Goto3/1, Digital Filter Design/1
  Packet Input1/1 -> Data Type Conversion1/1
  Packet Input1/3 -> Terminator1/1  "data error"
  Selector8/1 -> RT3/1
  Add10/1 -> Mux2/1
  Constant40/1 -> Add10/2
  Gain6/1 -> Add10/1
  Mux2/1 -> vicon measure/1

== system controller14/archived ==
  note: Vicon Input (single rigid body) not in use
  Data Type Conversion : DataTypeConversion  Commented=on  OutDataTypeStr=double  SaturateOnIntegerOverflow=off  RndMeth=Floor
  Gain7 : Gain  Commented=on  Gain=1/mdl.vicon.gain
  Gain8 : Gain  Commented=on  Gain=0.001
  Goto9 : Goto  Commented=on  GotoTag=vicon_measure
  Mux : Mux  Commented=on  Inputs=2
  Packet Input : sldrtlib/Packet Input  Commented=on  SampleTime=1/2000  MaxMissedTicks=100  ShowMissedTicks=off  YieldWhenWaiting=off  DrvName=Standard_Devices/UDP_Protocol  DrvAddress=18000  DrvOptions=[0 18385 49 57 50 46 49 54 56 46 49 54 56 46 49 52 54 0 0 0 0 0 0 0 0 0 0 0 0 0 0 0 0 0 0 0 0 0 0 0 0 0 0 0 0 0 0 0 0 0 0 0 0 0 0 0 0 0 0 0 0 0 0 0 0 0 0 0 0 0 0 0 0 0 0 0 0 0 0 0 0 0 0 0 0 0 0 0 0 0 0 0 0 0 0 0 0 0 0 0 0 0 0 0 0 0 0 0 0 0 0 0 0 0 0 0 0 0 0 0 0 0 0 0 0 0 0 0 0 0 0 0 0 0 0 0 0 0 0 0 0 0 0 0 0 0 0 0 0 0 0 0 0 0 0 0 0 0 0 0 0 0 0 0 0 0 0 0 0 0 0 0 0 0 0 0 0 0 0 0 0 0 0 0 0 0 0 0 0 0 0 0 0 0 0 0 0 0 0 0 0 0 0 0 0 0 0 0 0 0 0 0 0 0 0 0 0 0 0 0 0 0 0 0 0 0 0 0 0 0 0 0 0 0 0 0 0 0 0 0 0 0 0 0 0 0 0 0 0 0 0 0 0 0 0 0]  PacketSize=24  DataTypes='6*int32'  ShowReady=on  ShowError=on  PacketID=1  ByteOrder=2  ShowTimestamp=off
      settings: AttributesFormatString=UDP Protocol [18000]
  Selector2 : Selector  Commented=on  InputPortWidth=6  IndexOptions=Index vector (dialog)  Indices=[1:3]  OutputSizes=1
  Selector3 : Selector  Commented=on  InputPortWidth=6  IndexOptions=Index vector (dialog)  Indices=[4:6]  OutputSizes=1
  Terminator11 : Terminator  Commented=on
  data ready : Scope  Commented=on
  wires:
  Packet Input/2 -> data ready/1  "data ready"
  Gain8/1 -> Mux/1
  Gain7/1 -> Selector3/1, Selector2/1
  Mux/1 -> Goto9/1
  Selector2/1 -> Gain8/1
  Data Type Conversion/1 -> Gain7/1
  Selector3/1 -> Mux/2
  Packet Input/3 -> Terminator11/1  "data error"
  Packet Input/1 -> Data Type Conversion/1

== system controller14/back mapping from sat volt to torque-thrust ==
  sat_voltages : Inport
  Demux5 : Demux
  Digital Filter Design2 : dspfdesign/Digital Filter Design  mwdsp_browser_bugfix_var=off
  Mux10 : Mux
  Nemo Bee 1 : Lookup_n-D  NumberOfTableDimensions=1  BreakpointsForDimension1=lut.v4  Table=lut.T4  InternalRulePriority=Speed  RndMeth=Simplest
  Nemo Bee 2 : Lookup_n-D  NumberOfTableDimensions=1  BreakpointsForDimension1=lut.v1  Table=lut.T1  InternalRulePriority=Speed  RndMeth=Simplest
  Nemo Bee 3 : Lookup_n-D  NumberOfTableDimensions=1  BreakpointsForDimension1=lut.v3  Table=lut.T3  InternalRulePriority=Speed  RndMeth=Simplest
  Nemo Bee 4 : Lookup_n-D  NumberOfTableDimensions=1  BreakpointsForDimension1=lut.v2  Table=lut.T2  InternalRulePriority=Speed  RndMeth=Simplest
  Saturation{6..9} (4 alike) : Saturate  UpperLimit=1000  LowerLimit=0
  Scope : Scope  NumInputPorts=2
  Scope1 : Scope  Commented=on
  power_distribution_1 : MATLAB Function  TreatAsAtomicUnit=on
  torque_thrust : Outport
  wires:
  Saturation9/1 -> Mux10/4
  Saturation7/1 -> Mux10/2
  Nemo Bee 1/1 -> Saturation9/1
  Demux5/3 -> Nemo Bee 3/1
  Demux5/1 -> Nemo Bee 2/1
  Nemo Bee 2/1 -> Saturation6/1
  Demux5/4 -> Nemo Bee 1/1
  Saturation8/1 -> Mux10/3
  Nemo Bee 4/1 -> Saturation7/1
  Saturation6/1 -> Mux10/1
  Nemo Bee 3/1 -> Saturation8/1
  Demux5/2 -> Nemo Bee 4/1
  sat_voltages/1 -> Demux5/1
  power_distribution_1/1(torque_thrust) -> Scope1/1, torque_thrust/1
  Mux10/1 -> Digital Filter Design2/1, Scope/1  "sat motor thrust (mgf)"
  Digital Filter Design2/1 -> power_distribution_1/1(motor_thrust), Scope/2

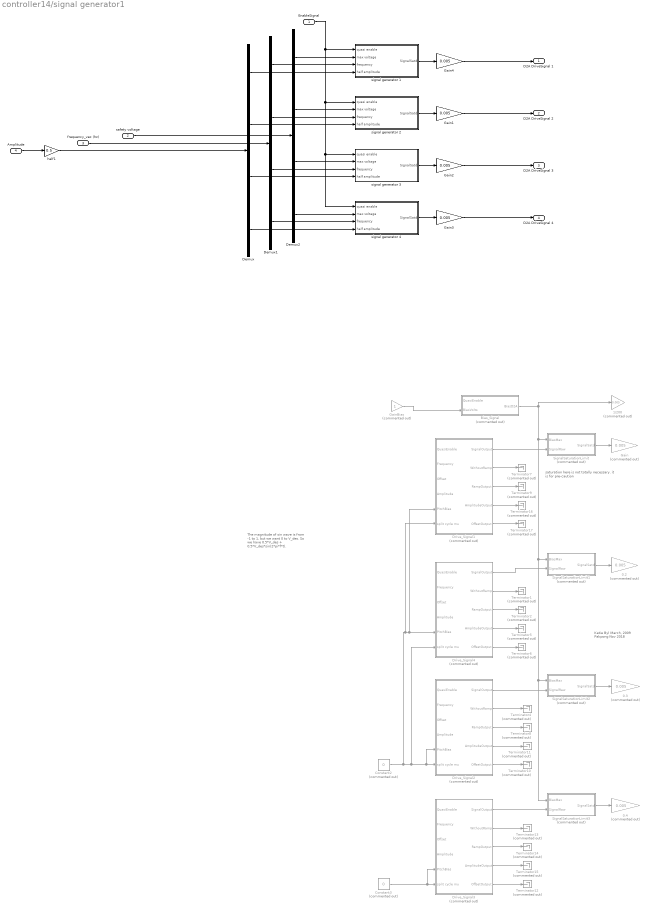
== system controller14/signal generator1 ==
  note: The magnitude of sin wave is from -1 to 1, but we want 0 to V_des. So we have 0.5*V_des + 0.5*V_des*sin(2*pi*f*t).
  note: Katie Byl
      | March, 2009
      |
      | Pakpong
      | Nov 2018
  note: saturation here is not totally necessary.
      | it is for pre-caution
  EnableSignal : Inport
  safety voltage : Inport  Port=2
  frequency_vec (hz) : Inport  Port=3
  Amplitude : Inport  Port=4
  0.2 : Gain  Commented=on  Gain=0.005
  0.3 : Gain  Commented=on  Gain=0.005
  0.4 : Gain  Commented=on  Gain=0.005
  1/200 : Gain  Commented=on  Gain=0.005
  Bias_Signal : Subsystem  Commented=on
  Constant2 : Constant  Commented=on  Value=0
  Constant3 : Constant  Commented=on  Value=0
  Demux : Demux
  Demux1 : Demux
  Demux2 : Demux
  Drive_Signal1 : Subsystem  Commented=on
  Drive_Signal2 : Subsystem  Commented=on
  Drive_Signal3 : Subsystem  Commented=on
  Drive_Signal4 : Subsystem  Commented=on
  Gain : Gain  Commented=on  Gain=0.005
  Gain{1..4} (4 alike) : Gain  Gain=0.005
  GainBias : Gain  Commented=on
  SignalSaturationLimit : Subsystem  Commented=on
  SignalSaturationLimit1 : Subsystem  Commented=on
  SignalSaturationLimit2 : Subsystem  Commented=on
  SignalSaturationLimit3 : Subsystem  Commented=on
  Terminator{1..2,4..17} (16 alike) : Terminator  Commented=on
  half1 : Gain  Gain=0.5
  signal generator 1 : Subsystem
  signal generator 2 : Subsystem
  signal generator 3 : Subsystem
  signal generator 4 : Subsystem
  D2A DriveSignal 1 : Outport
  D2A DriveSignal 2 : Outport  Port=2
  D2A DriveSignal 3 : Outport  Port=3
  D2A DriveSignal 4 : Outport  Port=4
  wires:
  Bias_Signal/1(BiasD2A) -> 1/200/1, SignalSaturationLimit3/1(BiasMax), SignalSaturationLimit2/1(BiasMax), SignalSaturationLimit1/1(BiasMax), SignalSaturationLimit/1(BiasMax)
  EnableSignal/1 -> signal generator 4/1(quasi enable), signal generator 3/1(quasi enable), signal generator 2/1(quasi enable), signal generator 1/1(quasi enable)
  SignalSaturationLimit/1(SignalSatd) -> Gain/1
  GainBias/1 -> Bias_Signal/2(BiasVolts)
  SignalSaturationLimit1/1(SignalSatd) -> 0.2/1
  Amplitude/1 -> half1/1
  Drive_Signal3/4(AmplitudeOutput) -> Terminator15/1
  Drive_Signal3/2(WithoutRamp) -> Terminator13/1
  Drive_Signal3/3(RampOutput) -> Terminator14/1
  Drive_Signal3/5(OffsetOutput) -> Terminator12/1
  Drive_Signal2/3(RampOutput) -> Terminator8/1
  Drive_Signal2/4(AmplitudeOutput) -> Terminator11/1
  Drive_Signal3/1(SignalOutput) -> SignalSaturationLimit3/2(SignalRaw)
  Drive_Signal2/5(OffsetOutput) -> Terminator10/1
  Drive_Signal2/2(WithoutRamp) -> Terminator4/1
  Demux/3 -> signal generator 3/4(half amplitude)
  Demux/4 -> signal generator 4/4(half amplitude)
  Constant2/1 -> Drive_Signal1/6(split cycle mu), Drive_Signal1/5(PitchBias), Drive_Signal4/5(PitchBias), Drive_Signal4/6(split cycle mu), Drive_Signal2/5(PitchBias), Drive_Signal2/6(split cycle mu)
  Constant3/1 -> Drive_Signal3/5(PitchBias), Drive_Signal3/6(split cycle mu)
  SignalSaturationLimit2/1(SignalSatd) -> 0.3/1
  SignalSaturationLimit3/1(SignalSatd) -> 0.4/1
  Drive_Signal2/1(SignalOutput) -> SignalSaturationLimit2/2(SignalRaw)
  half1/1 -> Demux/1
  frequency_vec (hz)/1 -> Demux1/1
  Demux1/1 -> signal generator 1/3(frequency)
  Demux1/2 -> signal generator 2/3(frequency)
  Demux1/3 -> signal generator 3/3(frequency)
  Demux1/4 -> signal generator 4/3(frequency)
  Drive_Signal4/1(SignalOutput) -> SignalSaturationLimit1/2(SignalRaw)
  Drive_Signal4/2(WithoutRamp) -> Terminator1/1
  Drive_Signal4/3(RampOutput) -> Terminator2/1
  Drive_Signal4/4(AmplitudeOutput) -> Terminator5/1
  Drive_Signal4/5(OffsetOutput) -> Terminator6/1
  Drive_Signal1/4(AmplitudeOutput) -> Terminator16/1
  Drive_Signal1/1(SignalOutput) -> SignalSaturationLimit/2(SignalRaw)
  Drive_Signal1/2(WithoutRamp) -> Terminator7/1
  Drive_Signal1/5(OffsetOutput) -> Terminator17/1
  Drive_Signal1/3(RampOutput) -> Terminator9/1
  Demux/1 -> signal generator 1/4(half amplitude)
  Demux/2 -> signal generator 2/4(half amplitude)
  signal generator 2/1(SignalSatd) -> Gain1/1
  signal generator 3/1(SignalSatd) -> Gain2/1
  signal generator 4/1(SignalSatd) -> Gain3/1
  signal generator 1/1(SignalSatd) -> Gain4/1
  Gain3/1 -> D2A DriveSignal 4/1
  Gain2/1 -> D2A DriveSignal 3/1
  Gain1/1 -> D2A DriveSignal 2/1
  Gain4/1 -> D2A DriveSignal 1/1
  safety voltage/1 -> Demux2/1
  Demux2/1 -> signal generator 1/2(max voltage)
  Demux2/2 -> signal generator 2/2(max voltage)
  Demux2/3 -> signal generator 3/2(max voltage)
  Demux2/4 -> signal generator 4/2(max voltage)

== system controller14/signal safety (no imag & NaN) ==
  In1 : Inport
  Complex to Real-Imag{,1..3} (4 alike) : ComplexToRealImag
  Constant{,1..3} (4 alike) : Constant  Value=0
  Demux : Demux
  IsNaN{,1..3} (4 alike) : RelationalOperator  Operator=isNaN  OutDataTypeStr=boolean  RndMeth=Simplest  InputSameDT=off
  Mux : Mux
  Switch{1..3,17} (4 alike) : Switch  Criteria=u2 > Threshold  SaturateOnIntegerOverflow=off  InputSameDT=off
  Terminator{,1..3} (4 alike) : Terminator
  Output : Outport
  wires:
  In1/1 -> Demux/1
  IsNaN/1 -> Switch17/2
  Constant/1 -> Switch17/1
  Switch17/1 -> Complex to Real-Imag/1
  Complex to Real-Imag/2 -> Terminator/1
  Demux/1 -> Switch17/3, IsNaN/1
  Complex to Real-Imag1/2 -> Terminator1/1
  Complex to Real-Imag1/1 -> Mux/2
  IsNaN1/1 -> Switch1/2
  Switch1/1 -> Complex to Real-Imag1/1
  Demux/2 -> Switch1/3, IsNaN1/1
  Constant1/1 -> Switch1/1
  Complex to Real-Imag2/2 -> Terminator2/1
  Complex to Real-Imag2/1 -> Mux/3
  IsNaN2/1 -> Switch2/2
  Switch2/1 -> Complex to Real-Imag2/1
  Demux/3 -> Switch2/3, IsNaN2/1
  Constant2/1 -> Switch2/1
  Complex to Real-Imag3/2 -> Terminator3/1
  Complex to Real-Imag3/1 -> Mux/4
  IsNaN3/1 -> Switch3/2
  Demux/4 -> IsNaN3/1, Switch3/3
  Switch3/1 -> Complex to Real-Imag3/1
  Constant3/1 -> Switch3/1
  Mux/1 -> Output/1
  Complex to Real-Imag/1 -> Mux/1

== system controller14/voltage safety (no imag & NaN) ==
  In1 : Inport
  Complex to Real-Imag{,1..3} (4 alike) : ComplexToRealImag
  Delay{,1..3} (4 alike) : Delay  DelayLength=1
  Demux : Demux
  IsNaN{,1..3} (4 alike) : RelationalOperator  Operator=isNaN  OutDataTypeStr=boolean  RndMeth=Simplest  InputSameDT=off
  Mux : Mux
  Switch{1..3,17} (4 alike) : Switch  Criteria=u2 > Threshold  SaturateOnIntegerOverflow=off  InputSameDT=off
  Terminator{,1..3} (4 alike) : Terminator
  Output : Outport
  wires:
  In1/1 -> Demux/1
  IsNaN/1 -> Switch17/2
  Switch17/1 -> Delay1/1, Complex to Real-Imag/1
  Complex to Real-Imag/2 -> Terminator/1
  Demux/1 -> Switch17/3, IsNaN/1
  Complex to Real-Imag1/2 -> Terminator1/1
  Complex to Real-Imag1/1 -> Mux/2
  IsNaN1/1 -> Switch1/2
  Switch1/1 -> Delay/1, Complex to Real-Imag1/1
  Demux/2 -> Switch1/3, IsNaN1/1
  Complex to Real-Imag2/2 -> Terminator2/1
  Complex to Real-Imag2/1 -> Mux/3
  IsNaN2/1 -> Switch2/2
  Switch2/1 -> Delay2/1, Complex to Real-Imag2/1
  Demux/3 -> Switch2/3, IsNaN2/1
  Complex to Real-Imag3/2 -> Terminator3/1
  Complex to Real-Imag3/1 -> Mux/4
  IsNaN3/1 -> Switch3/2
  Demux/4 -> IsNaN3/1, Switch3/3
  Switch3/1 -> Delay3/1, Complex to Real-Imag3/1
  Mux/1 -> Output/1
  Complex to Real-Imag/1 -> Mux/1
  Delay/1 -> Switch1/1
  Delay1/1 -> Switch17/1
  Delay2/1 -> Switch2/1
  Delay3/1 -> Switch3/1

== system controller14/Archived data for rerun/time1 ==
  constant : Constant
  time : DiscreteIntegrator  gainval=mdl.f_high  InitialCondition=1  SampleTime=mdl.T_high  UpperSaturationLimit=1  LowerSaturationLimit=0  ICPrevOutput=DiscIntNeverNeededParam  ICPrevScaledInput=DiscIntNeverNeededParam
  index : Outport
  wires:
  constant/1 -> time/1
  time/1 -> index/1

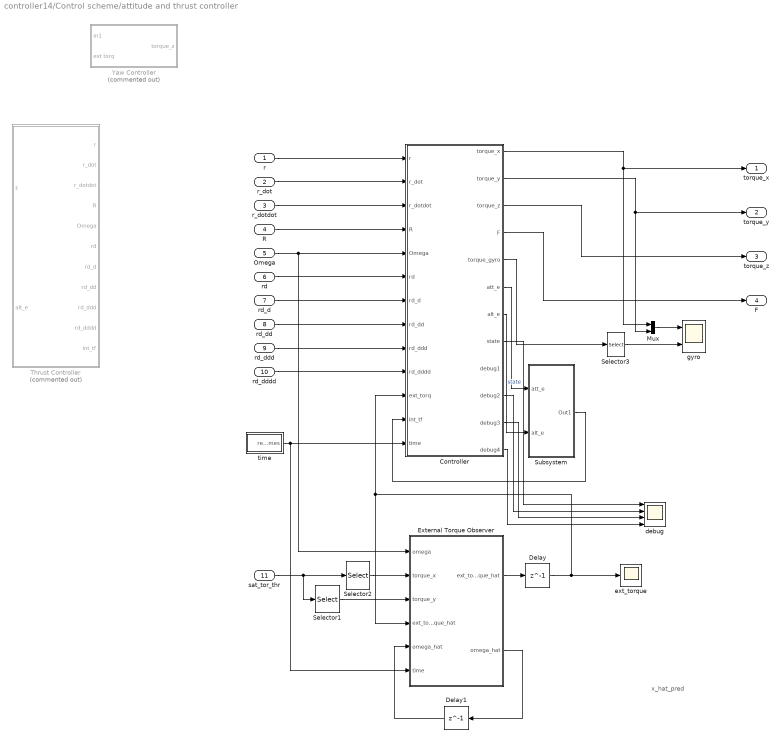
== system controller14/Control scheme/attitude and thrust controller ==
  note: x_hat_pred
  r : Inport
  r_dot : Inport  Port=2
  r_dotdot : Inport  Port=3
  R : Inport  Port=4
  Omega : Inport  Port=5
  rd : Inport  Port=6
  rd_d : Inport  Port=7
  rd_dd : Inport  Port=8
  rd_ddd : Inport  Port=9
  rd_dddd : Inport  Port=10
  sat_tor_thr : Inport  Port=11
  Controller : MATLAB Function  TreatAsAtomicUnit=on
  Delay : Delay  DelayLength=1  InitialCondition=ctr2.torque_obs.ext_torq_hat_init  SampleTime=mdl.T
  Delay1 : Delay  DelayLength=1  InitialCondition=ctr2.torque_obs.omega_hat_init  SampleTime=mdl.T
  External Torque Observer : MATLAB Function  TreatAsAtomicUnit=on
  Mux : Mux  Inputs=2
  Selector1 : Selector  InputPortWidth=4  IndexOptions=Index vector (dialog)  Indices=[2]  OutputSizes=1
  Selector2 : Selector  InputPortWidth=4  IndexOptions=Index vector (dialog)  Indices=[1]  OutputSizes=1
  Selector3 : Selector  InputPortWidth=3  IndexOptions=Index vector (dialog)  Indices=[1 2]  OutputSizes=1
  Subsystem : Subsystem
  Thrust Controller : MATLAB Function  Commented=on  TreatAsAtomicUnit=on
  Yaw Controller : Subsystem  Commented=on
  debug : Scope  NumInputPorts=4
  ext_torque : Scope
  gyro : Scope  NumInputPorts=2
  time : Subsystem
  torque_x : Outport
  torque_y : Outport  Port=2
  torque_z : Outport  Port=3
  F : Outport  Port=4
  wires:
  r/1 -> Controller/1(r)
  Controller/1(torque_x) -> torque_x/1, Mux/1
  r_dot/1 -> Controller/2(r_dot)
  r_dotdot/1 -> Controller/3(r_dotdot)
  R/1 -> Controller/4(R)
  Controller/2(torque_y) -> torque_y/1, Mux/2
  Omega/1 -> External Torque Observer/1(omega), Controller/5(Omega)
  rd/1 -> Controller/6(rd)
  rd_d/1 -> Controller/7(rd_d)
  rd_dd/1 -> Controller/8(rd_dd)
  rd_ddd/1 -> Controller/9(rd_ddd)
  rd_dddd/1 -> Controller/10(rd_dddd)
  Controller/3(torque_z) -> torque_z/1
  External Torque Observer/2(omega_hat) -> Delay1/1
  Delay/1 -> ext_torque/1, External Torque Observer/4("ext_torque_hat "), Controller/11(ext_torq)
  External Torque Observer/1(ext_torque_hat) -> Delay/1
  Delay1/1 -> External Torque Observer/5("omega_hat ")
  time/1(real times) -> External Torque Observer/6(time), Controller/13(time)
  Subsystem/1(Out1) -> Controller/12(int_tf)
  Controller/6(att_e) -> Subsystem/1(att_e)
  Selector2/1 -> External Torque Observer/2(torque_x)
  Selector1/1 -> External Torque Observer/3(torque_y)
  sat_tor_thr/1 -> Selector2/1, Selector1/1
  Controller/7(alt_e) -> Subsystem/2(alt_e)
  Controller/4(F) -> F/1
  Mux/1 -> gyro/1
  Selector3/1 -> gyro/2
  Controller/5(torque_gyro) -> Selector3/1
  Controller/8(state) -> debug/1  "state"
  Controller/10(debug2) -> debug/2
  Controller/11(debug3) -> debug/3
  Controller/12(debug4) -> debug/4

== system controller14/Control scheme/observer ==
  xyz : Inport
  euler : Inport  Port=2
  Rotaion : Subsystem
  lateral observer : Subsystem
  r : Outport
  r_dot : Outport  Port=2
  r_dotdot : Outport  Port=3
  R : Outport  Port=4
  Omega : Outport  Port=5
  Rdot : Outport  Port=6
  wires:
  lateral observer/1(r) -> r/1
  xyz/1 -> lateral observer/1(XYZ)
  lateral observer/2(r_dot) -> r_dot/1
  lateral observer/3(r_dotdot) -> r_dotdot/1
  Rotaion/1(R) -> R/1
  euler/1 -> Rotaion/1(Euler)
  Rotaion/2(Rdot) -> Rdot/1
  Rotaion/3(Omega) -> Omega/1

== system controller14/Control scheme/time ==
  constant : Constant
  time : DiscreteIntegrator  gainval=1  SampleTime=-1  UpperSaturationLimit=1  LowerSaturationLimit=0  ICPrevOutput=DiscIntNeverNeededParam  ICPrevScaledInput=DiscIntNeverNeededParam
  real times : Outport
  wires:
  constant/1 -> time/1
  time/1 -> real times/1

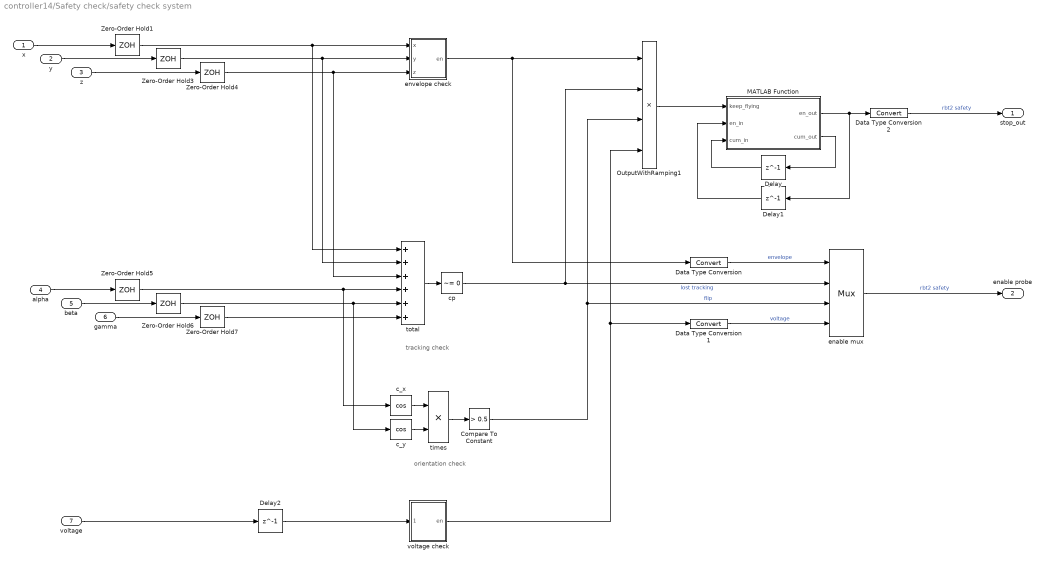
== system controller14/Safety check/safety check system ==
  note: orientation check
  note: tracking check
  x : Inport
  y : Inport  Port=2
  z : Inport  Port=3
  alpha : Inport  Port=4
  beta : Inport  Port=5
  gamma : Inport  Port=6
  voltage : Inport  Port=7
  Compare To Constant : simulink/Logic and Bit Operations/Compare To Constant  relop=>  const=0.5  OutDataTypeStr=uint8
  Data Type Conversion : DataTypeConversion  SaturateOnIntegerOverflow=off  RndMeth=Floor
  Data Type Conversion1 : DataTypeConversion  SaturateOnIntegerOverflow=off  RndMeth=Floor
  Data Type Conversion2 : DataTypeConversion  SaturateOnIntegerOverflow=off  RndMeth=Floor
  Delay : Delay  DelayLength=1
  Delay1 : Delay  DelayLength=1  InitialCondition=1
  Delay2 : Delay  DelayLength=1  InitialCondition=zeros(4,1)
  MATLAB Function : MATLAB Function  TreatAsAtomicUnit=on  SystemSampleTime=mdl.T
  OutputWithRamping1 : Product  Inputs=4  RndMeth=Zero
  Zero-Order Hold{1,3..7} (6 alike) : ZeroOrderHold  SampleTime=mdl.T
  c_x : Trigonometry  Operator=cos
  c_y : Trigonometry  Operator=cos
  cp : simulink/Logic and Bit Operations/Compare To Zero  relop=~=  OutDataTypeStr=uint8
  enable mux : Mux
      settings: DisplayOption=signals
  envelope check : MATLAB Function  TreatAsAtomicUnit=on
  times : Product  RndMeth=Zero
  total : Sum  Inputs=++++++
  voltage check : MATLAB Function  TreatAsAtomicUnit=on
  stop_out : Outport
  enable probe : Outport  Port=2
  wires:
  y/1 -> Zero-Order Hold3/1
  cp/1 -> enable mux/2, OutputWithRamping1/2  "lost tracking"
  envelope check/1(en) -> Data Type Conversion/1, OutputWithRamping1/1
  enable mux/1 -> enable probe/1  "rbt2 safety"
  Data Type Conversion/1 -> enable mux/1  "envelope"
  times/1 -> Compare To Constant/1
  voltage check/1(en) -> OutputWithRamping1/4, Data Type Conversion1/1
  z/1 -> Zero-Order Hold4/1
  Compare To Constant/1 -> OutputWithRamping1/3, enable mux/3  "flip"
  total/1 -> cp/1
  x/1 -> Zero-Order Hold1/1
  alpha/1 -> Zero-Order Hold5/1
  beta/1 -> Zero-Order Hold6/1
  c_x/1 -> times/1
  c_y/1 -> times/2
  Data Type Conversion1/1 -> enable mux/4  "voltage"
  voltage/1 -> Delay2/1
  gamma/1 -> Zero-Order Hold7/1
  OutputWithRamping1/1 -> MATLAB Function/1(keep_flying)
  Delay1/1 -> MATLAB Function/2(en_in)
  MATLAB Function/1(en_out) -> Delay1/1, Data Type Conversion2/1
  Delay/1 -> MATLAB Function/3(cum_in)
  MATLAB Function/2(cum_out) -> Delay/1
  Data Type Conversion2/1 -> stop_out/1  "rbt2 safety"
  Delay2/1 -> voltage check/1(voltage)
  Zero-Order Hold1/1 -> total/1, envelope check/1(x)
  Zero-Order Hold3/1 -> envelope check/2(y), total/2
  Zero-Order Hold4/1 -> total/3, envelope check/3(z)
  Zero-Order Hold5/1 -> total/4, c_x/1
  Zero-Order Hold6/1 -> total/5, c_y/1
  Zero-Order Hold7/1 -> total/6
